simulink model "ASK"  (R2021b)
settings: Solver=VariableStepAuto  StartTime=0.0  StopTime=5  RelTol=1e-3
libraries: simulink x1, commutil2 x1, dspsigops x1, dspquant2 x1
settings Model: Creator=shankar  LastModifiedBy=ZephyrY
settings SolverCC: AlgebraicLoopSolver=TrustRegion
settings DebuggingCC: SFMachineParentedDataDiag=warning

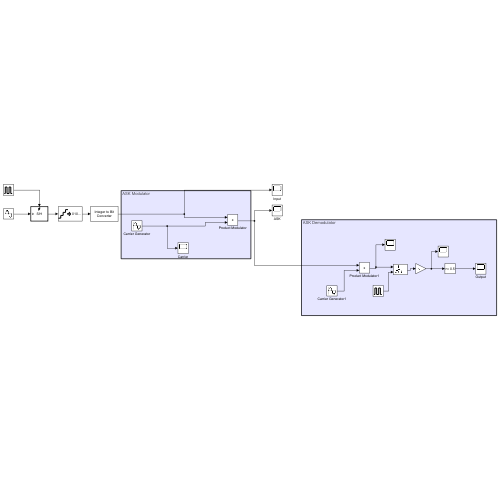
[thumbnail: Simulink's stored preview of the top-level diagram]
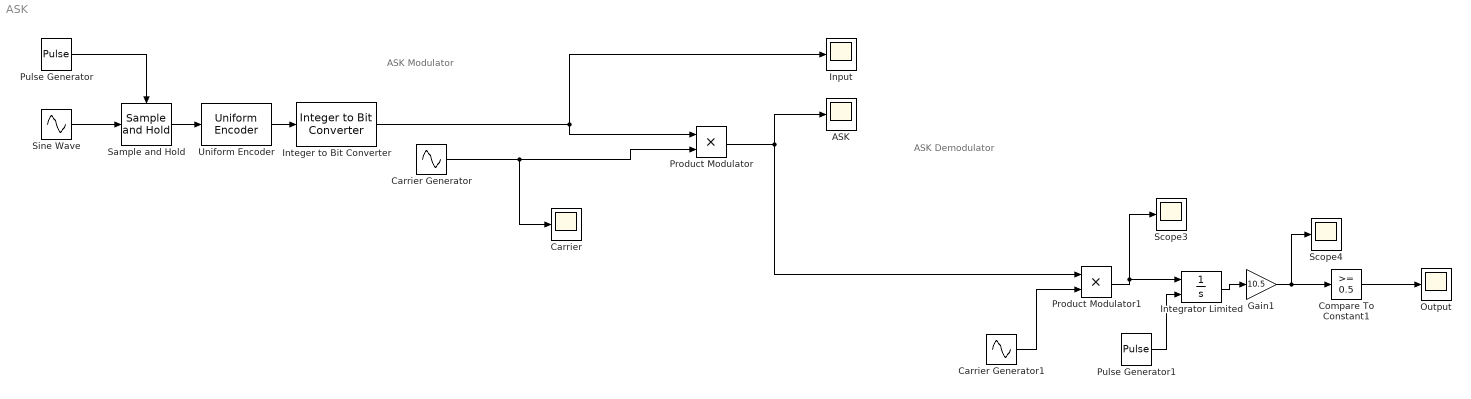
== system ASK ==
  note: ASK Demodulator
  note: ASK Modulator
  ASK : Scope
  Carrier : Scope
  Carrier Generator : Sin  Frequency=2*3.141*10  SampleTime=1e-5
  Carrier Generator1 : Sin  Frequency=2*3.141*10  SampleTime=1e-5
  Compare To Constant1 : simulink/Logic and Bit Operations/Compare To Constant  relop=>=  const=0.5  OutDataTypeStr=boolean
  Gain1 : Gain  Gain=10.5
  Input : Scope
  Integer to Bit Converter : commutil2/Integer to Bit Converter  nbits=2  signedInputValues=Signed  bitOrder=MSB first  outDtype=Inherit via internal rule
  Integrator Limited : Integrator  ExternalReset=rising  LimitOutput=on  UpperSaturationLimit=0.08  LowerSaturationLimit=0  WrappedStateUpperValue=0.1  WrappedStateLowerValue=-0.1
  Output : Scope
  Product Modulator : Product
  Product Modulator1 : Product
  Pulse Generator : DiscretePulseGenerator  PulseType=Time based  Period=0.5  PulseWidth=20
  Pulse Generator1 : DiscretePulseGenerator  PulseType=Time based  Period=0.5  PulseWidth=20
  Sample and Hold : dspsigops/Sample and Hold  trig=Rising edge  initCond=0  latchinput=off
  Scope3 : Scope
  Scope4 : Scope
  Sine Wave : Sin  Frequency=2*pi*1  SampleTime=1e-5
  Uniform Encoder : dspquant2/Uniform Encoder  peak=1  bits=2  otype=Signed integer
  wires:
  Carrier Generator/1 -> Carrier/1, Product Modulator/2
  Product Modulator/1 -> Product Modulator1/1, ASK/1
  Integer to Bit Converter/1 -> Product Modulator/1, Input/1
  Product Modulator1/1 -> Scope3/1, Integrator Limited/1
  Carrier Generator1/1 -> Product Modulator1/2
  Integrator Limited/1 -> Gain1/1
  Gain1/1 -> Scope4/1, Compare To Constant1/1
  Compare To Constant1/1 -> Output/1
  Sample and Hold/1 -> Uniform Encoder/1
  Uniform Encoder/1 -> Integer to Bit Converter/1
  Sine Wave/1 -> Sample and Hold/1
  Pulse Generator/1 -> Sample and Hold/Trigger
  Pulse Generator1/1 -> Integrator Limited/2
